simulink model "Li_Battry_reload"  (R2024b)
settings: Solver=VariableStepAuto  StartTime=0.0  StopTime=10.0  RelTol=1e-3
undefined symbols (not defined in the file): Ion, Lithium
libraries: spsControlledCurrentSourceLib x2, spsIdealSwitchLib x2, spsBatteryLib x1, spsVoltageMeasurementLib x1, sps_lib x1
settings Model: Creator=王翘楚  LastModifiedBy=Administrator

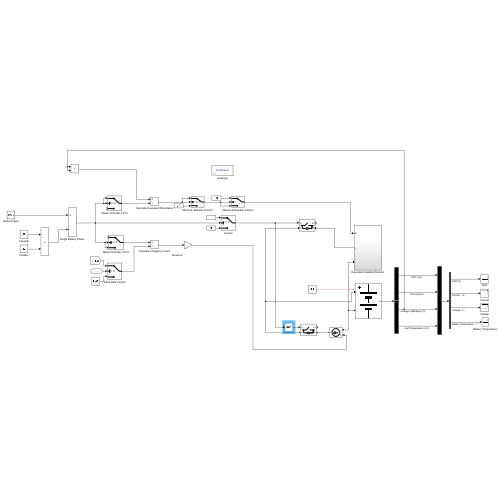
[thumbnail: Simulink's stored preview of the top-level diagram]
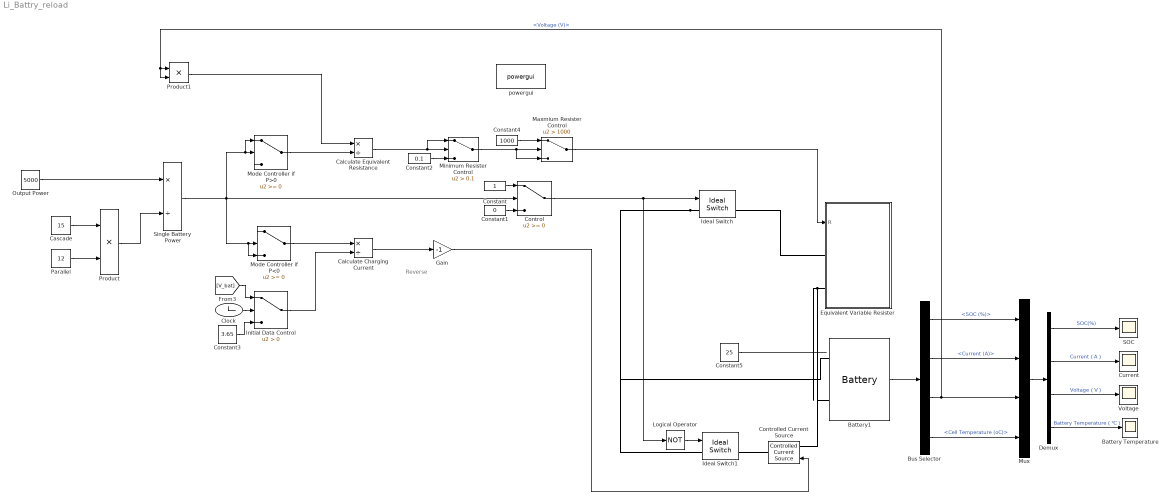
== system Li_Battry_reload ==
  note: Reverse
  Battery Temperature : Scope
  Battery1 : spsBatteryLib/Battery  BatType=Lithium-Ion  NomV=3.2  NomQ=5  SOC=100  Batt_Tr=1  PresetModel=off  MaxQ=5  MinV=2.5  FullV=3.65  Dis_rate=2.1739  R=0.0064  Normal_OP=4.5217  expZone="[3.4572     0.24565]"
      settings: LibrarySourceBlock=electricdrivelib/Extra Sources/Battery
  Bus Selector : BusSelector  OutputSignals=SOC (%),Current (A),Voltage (V),Cell Temperature (oC)
  Calculate Charging Current : Product  Inputs=*/
  Calculate Equivalent Resistance : Product  Inputs=*/
  Cascade : Constant  Value=15  VectorParams1D=off
  Clock : Clock
  Constant : Constant
  Constant1 : Constant  Value=0
  Constant2 : Constant  Value=0.1
  Constant3 : Constant  Value=3.65
  Constant4 : Constant  Value=1000
  Constant5 : Constant  Value=25
  Control : Switch  SaturateOnIntegerOverflow=off  InputSameDT=off
  Controlled Current Source : spsControlledCurrentSourceLib/Controlled Current Source  Initialize=on  Source_Type=AC  Amplitude=0  Phase=0  Frequency=0  Measurements=None
  Current : Scope
  Demux : Demux
  Equivalent Variable Resister : Subsystem
  Gain : Gain  Gain=-1
  Ideal Switch : spsIdealSwitchLib/Ideal Switch  Ron=0.001  Lon=0  IC=0  Rs=1e5  Cs=inf  Measurements=on
  Ideal Switch1 : spsIdealSwitchLib/Ideal Switch  Ron=0.001  Lon=0  IC=0  Rs=1e5  Cs=inf  Measurements=on
  Initial Data Control : Switch  Criteria=u2 > Threshold  SaturateOnIntegerOverflow=off  InputSameDT=off
  Logical Operator : Logic  Operator=NOT  AllPortsSameDT=off  OutDataTypeStr=boolean
  Maxmium Resister Control : Switch  Criteria=u2 > Threshold  Threshold=1000  SaturateOnIntegerOverflow=off  InputSameDT=off
  Minimum Resister Control : Switch  Criteria=u2 > Threshold  Threshold=0.1  SaturateOnIntegerOverflow=off  InputSameDT=off
  Mode Controller if P<0 : Switch  SaturateOnIntegerOverflow=off  InputSameDT=off
  Mode Controller if P>0 : Switch  SaturateOnIntegerOverflow=off  InputSameDT=off
  Mux : Mux
  Output Power : Constant  Value=5000
  Parallel : Constant  Value=12
  Product : Product
  Product1 : Product
  SOC : Scope
  Single Battery Power : Product  Inputs=*/
  Voltage : Scope
  powergui : sps_lib/powergui  Priority=1  SimulationMode=Continuous  SampleTime=50e-6  frequency=60  Iterations=50  frequencyindice=0  Pbase=100e6  ErrMax=1e-4  UnitsV=kV  UnitsW=MW  buscounter=0  FunctionMessages=off  echomessages=off  EnableUseOfTLC=off  CurrentSourceSwitches=off  DisableSnubberDevices=off  DisableRonSwitches=off  DisableVfSwitches=off  DisplayEquations=off  AutomaticDiscreteSolvers=off  SolverType=Tustin/Backward Euler (TBE)  Interpol=off  ExternalGateDelay=off  methode=off  Ts=100  x0status=blocks  SPID=on  SwTol=0  HookPort=off  NonlinearTolerance=1e-4  nMaxIteration=100  ContinueOnMaxIteration=off  RestoreLinks=warning  ResistiveCurrentMeasurement=off  Frange=[0:2:500]  Ylog=off  Xlog=on  ShowGrid=off  save=off  variable=ZData  structure=0  ZoomFFT=off  StartTime=0.0  cycles=1  DisplayStyle=1  fundamental=60  FreqAxis=off  MaxFrequency=1000  frequencyindicesteady=1  RmsSteady=1  display=off
  wires:
  Initial Data Control/1 -> Calculate Charging Current/2
  Calculate Charging Current/1 -> Gain/1
  Minimum Resister Control/1 -> Maxmium Resister Control/3, Maxmium Resister Control/2
  Mode Controller if P>0/1 -> Calculate Equivalent Resistance/2
  Constant3/1 -> Initial Data Control/3
  [V_bat] -> Initial Data Control/1
  Parallel/1 -> Product/2
  Constant4/1 -> Maxmium Resister Control/1
  Clock/1 -> Initial Data Control/2
  Output Power/1 -> Single Battery Power/1
  Product/1 -> Single Battery Power/2
  Mode Controller if P<0/1 -> Calculate Charging Current/1
  Constant2/1 -> Minimum Resister Control/3
  Cascade/1 -> Product/1
  Product1/1 -> Calculate Equivalent Resistance/1
  Calculate Equivalent Resistance/1 -> Minimum Resister Control/1, Minimum Resister Control/2
  Demux/1 -> SOC/1  "SOC(%)"
  Bus Selector/3 -> Product1/2, Product1/1, Mux/3  "<Voltage (V)>"
  Demux/4 -> Battery Temperature/1  "Battery Temperature（℃）"
  Maxmium Resister Control/1 -> Equivalent Variable Resister/1(R)
  Demux/3 -> Voltage/1  "Voltage（V）"
  Battery1/1 -> Bus Selector/1
  Demux/2 -> Current/1  "Current（A）"
  Single Battery Power/1 -> Mode Controller if P>0/1, Mode Controller if P>0/2, Control/2, Mode Controller if P<0/3, Mode Controller if P<0/2
  Bus Selector/1 -> Mux/1  "<SOC (%)>"
  Bus Selector/4 -> Mux/4  "<Cell Temperature (oC)>"
  Mux/1 -> Demux/1
  Control/1 -> Ideal Switch/1, Logical Operator/1
  Constant/1 -> Control/1
  Constant5/1 -> ?
  Bus Selector/2 -> Mux/2  "<Current (A)>"
  Constant1/1 -> Control/3
  Logical Operator/1 -> Ideal Switch1/1
  Gain/1 -> Controlled Current Source/1
  connections:
  Equivalent Variable Resister/LConn2 -- Controlled Current Source/LConn1 -- Battery1/LConn2
  Ideal Switch/LConn1 -- Ideal Switch1/LConn1 -- Battery1/LConn1
  Controlled Current Source/RConn1 -- Ideal Switch1/RConn1
  Ideal Switch/RConn1 -- Equivalent Variable Resister/LConn1

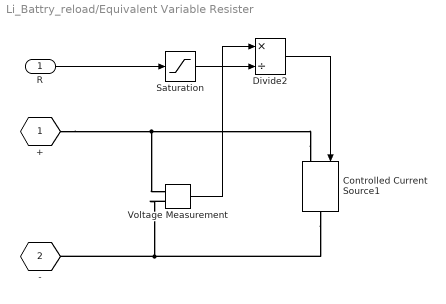
== system Li_Battry_reload/Equivalent Variable Resister ==
  R : Inport
  Controlled Current Source1 : spsControlledCurrentSourceLib/Controlled Current Source  Initialize=on  Source_Type=AC  Amplitude=0  Phase=0  Frequency=0  Measurements=None
  Divide2 : Product  Inputs=*/
  Saturation : Saturate  UpperLimit=1000  LowerLimit=0.1
  Voltage Measurement : spsVoltageMeasurementLib/Voltage Measurement  PhasorSimulation=off  OutputType=Complex  PSBequivalent=0
  + : PMIOPort  Tag=PMCPort  Side=Left
  - : PMIOPort  Tag=PMCPort  Port=2  Side=Left
  wires:
  Voltage Measurement/1 -> Divide2/1
  R/1 -> Saturation/1
  Saturation/1 -> Divide2/2
  Divide2/1 -> Controlled Current Source1/1
  connections:
  Controlled Current Source1/RConn1 -- -/RConn1 -- Voltage Measurement/LConn2
  Controlled Current Source1/LConn1 -- +/RConn1 -- Voltage Measurement/LConn1
